simulink library "slupdate_flipflops"  (Simulink 3.00)
libraries: simulink_extras x2
settings Model: Creator=mani  LastModifiedBy=mani

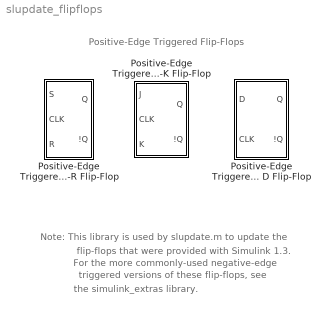
== system slupdate_flipflops ==
  note: Positive-Edge Triggered Flip-Flops
  note: Note: This library is used by slupdate.m to update the
  note: flip-flops that were provided with Simulink 1.3.
  note: For the more commonly-used negative-edge
  note: triggered versions of these flip-flops, see
  note: the simulink_extras library.
  Positive-Edge Triggered D Flip-Flop : Subsystem  mask(PosEdgeDFlipFlop){initial_condition=0}
      mask prompts: initial_condition "Initial Condition"
      mask help: D Flip-Flop Block (Positive Edge Triggered)
      mask init:
      | if ~any(initial_condition == [0 1])
      |   error('The initial condition has to be 0 or 1.');
      | end
  Positive-Edge Triggered J-K Flip-Flop : Subsystem  mask(PosEdgeJKFlipFlop){initial_condition=0}
      mask prompts: initial_condition "Initial Condition:"
      mask help: J-K Flip Flop Block (Positive Edge Triggered)
      mask init:
      | if ~any(initial_condition == [0 1])
      |   error('The initial condition has to be 0 or 1.');
      | end
  Positive-Edge Triggered S-R Flip-Flop : Subsystem  mask(PosEdgeSRFlipFlop){initial_condition=0}
      mask prompts: initial_condition "Initial condition:"
      mask help: S-R Flip Flop Block (Positive Edge Triggered)
      mask init:
      | if ~any(initial_condition == [0 1])
      |   error('The initial condition has to be 0 or 1.');
      | end

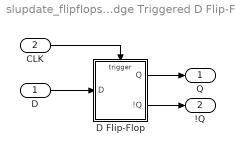
== system slupdate_flipflops/Positive-Edge Triggered D Flip-Flop ==
  D : Inport  Port=1  PortWidth=-1  SampleTime=-1  DataType=auto
      settings: SignalType=auto
  CLK : Inport  Port=2  PortWidth=-1  SampleTime=-1  DataType=auto
      settings: SignalType=auto
  D Flip-Flop : Subsystem
  Q : Outport  Port=1
  !Q : Outport  Port=2
  wires:
  CLK/1 -> D Flip-Flop/Trigger
  D/1 -> D Flip-Flop/1(D)
  D Flip-Flop/1(Q) -> Q/1
  D Flip-Flop/2(!Q) -> !Q/1

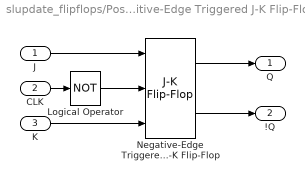
== system slupdate_flipflops/Positive-Edge Triggered J-K Flip-Flop ==
  J : Inport  Port=1  PortWidth=-1  SampleTime=-1  DataType=auto
      settings: SignalType=auto
  CLK : Inport  Port=2  PortWidth=-1  SampleTime=-1  DataType=auto
      settings: SignalType=auto
  K : Inport  Port=3  PortWidth=-1  SampleTime=-1  DataType=auto
      settings: SignalType=auto
  Logical Operator : Logic  Operator=NOT  Inputs=2
  Negative-Edge Triggered J-K Flip-Flop : simulink_extras/Flip Flops/J-K Flip-Flop  initial_condition=initial_condition
  Q : Outport  Port=1
  !Q : Outport  Port=2
  wires:
  Negative-Edge Triggered J-K Flip-Flop/2 -> !Q/1
  Negative-Edge Triggered J-K Flip-Flop/1 -> Q/1
  J/1 -> Negative-Edge Triggered J-K Flip-Flop/1
  K/1 -> Negative-Edge Triggered J-K Flip-Flop/3
  CLK/1 -> Logical Operator/1
  Logical Operator/1 -> Negative-Edge Triggered J-K Flip-Flop/2

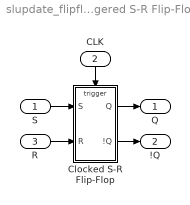
== system slupdate_flipflops/Positive-Edge Triggered S-R Flip-Flop ==
  S : Inport  Port=1  PortWidth=-1  SampleTime=-1  DataType=auto
      settings: SignalType=auto
  CLK : Inport  Orientation=down  Port=2  PortWidth=-1  SampleTime=-1  DataType=auto
      settings: SignalType=auto
  R : Inport  Port=3  PortWidth=-1  SampleTime=-1  DataType=auto
      settings: SignalType=auto
  Clocked S-R Flip-Flop : Subsystem
  Q : Outport  Port=1
  !Q : Outport  Port=2
  wires:
  Clocked S-R Flip-Flop/2(!Q) -> !Q/1
  R/1 -> Clocked S-R Flip-Flop/2(R)
  S/1 -> Clocked S-R Flip-Flop/1(S)
  Clocked S-R Flip-Flop/1(Q) -> Q/1
  CLK/1 -> Clocked S-R Flip-Flop/Trigger

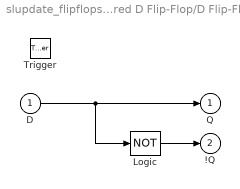
== system slupdate_flipflops/Positive-Edge Triggered D Flip-Flop/D Flip-Flop ==
  D : Inport  Port=1  PortWidth=-1  SampleTime=-1  DataType=auto
      settings: SignalType=auto
  Trigger : TriggerPort  TriggerType=rising  OutputDataType=auto
  Logic : Logic  Operator=NOT  Inputs=1
  Q : Outport  Port=1  InitialOutput=initial_condition
  !Q : Outport  Port=2  InitialOutput=~initial_condition
  wires:
  Logic/1 -> !Q/1
  D/1 -> Q/1, Logic/1

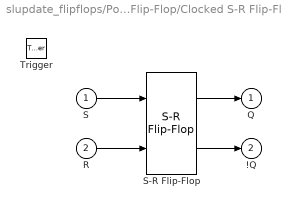
== system slupdate_flipflops/Positive-Edge Triggered S-R Flip-Flop/Clocked S-R Flip-Flop ==
  S : Inport  Port=1  PortWidth=-1  SampleTime=-1  DataType=auto
      settings: SignalType=auto
  R : Inport  Port=2  PortWidth=-1  SampleTime=-1  DataType=auto
      settings: SignalType=auto
  Trigger : TriggerPort  TriggerType=rising  OutputDataType=auto
  S-R Flip-Flop : simulink_extras/Flip Flops/S-R Flip-Flop  initial_condition=initial_condition
  Q : Outport  Port=1  InitialOutput=initial_condition
  !Q : Outport  Port=2  InitialOutput=~initial_condition
  wires:
  S-R Flip-Flop/2 -> !Q/1
  S-R Flip-Flop/1 -> Q/1
  R/1 -> S-R Flip-Flop/2
  S/1 -> S-R Flip-Flop/1
